simulink model "SimulinkModel"  (R2022b)
settings: Solver=FixedStepAuto  StartTime=0.0  StopTime=10.0  FixedStep=1e-06  RelTol=1e-3
settings Model: DataDictionary=BusSystem.sldd  Creator=cao2851  LastModifiedBy=cao2851

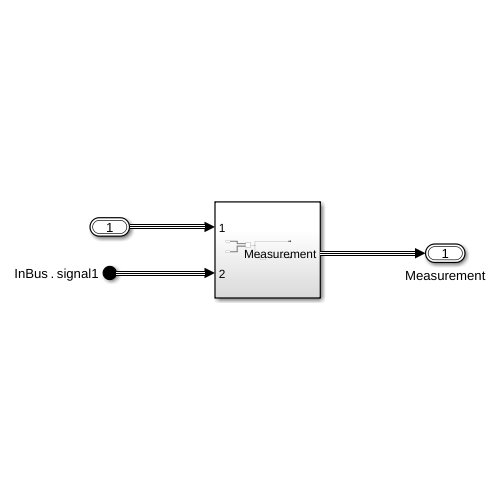
[thumbnail: Simulink's stored preview of the top-level diagram]
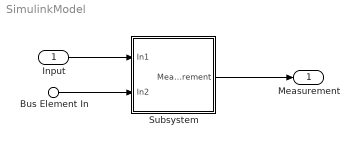
== system SimulinkModel ==
  Input : Inport  OutDataTypeStr=Bus: bus3
  Bus Element In : Inport  Port=2  PortName=InBus  Element=signal1
  Subsystem : Subsystem
  Measurement : Outport  OutDataTypeStr=Bus: slBus1
  wires:
  Input/1 -> Subsystem/1(In1)
  Bus Element In/1 -> Subsystem/2(In2)
  Subsystem/1(Measurement) -> Measurement/1

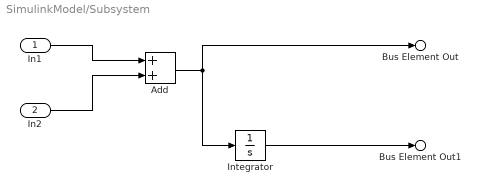
== system SimulinkModel/Subsystem ==
  In1 : Inport
  In2 : Inport  Port=2
  Add : Sum
  Integrator : Integrator
  Bus Element Out : Outport  PortName=Measurement  Element=add
  Bus Element Out1 : Outport  PortName=Measurement  Element=integrator
  wires:
  In1/1 -> Add/1
  In2/1 -> Add/2
  Integrator/1 -> Bus Element Out1/1
  Add/1 -> Integrator/1, Bus Element Out/1
